simulink model "DolphinDrone_backup"  (R2024b)
settings: Solver=ode4  StartTime=0.0  StopTime=120  FixedStep=0.001  RelTol=1e-3
libraries: slpidlib x3, aerolibobsolete x1, simulink x1
settings Model: Creator=limchanyeong  LastModifiedBy=limchanyeong

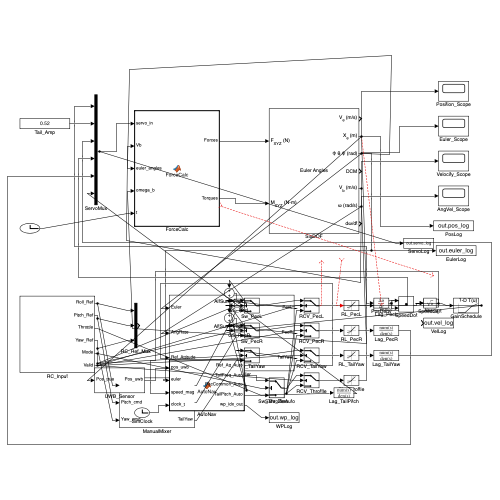
[thumbnail: Simulink's stored preview of the top-level diagram]
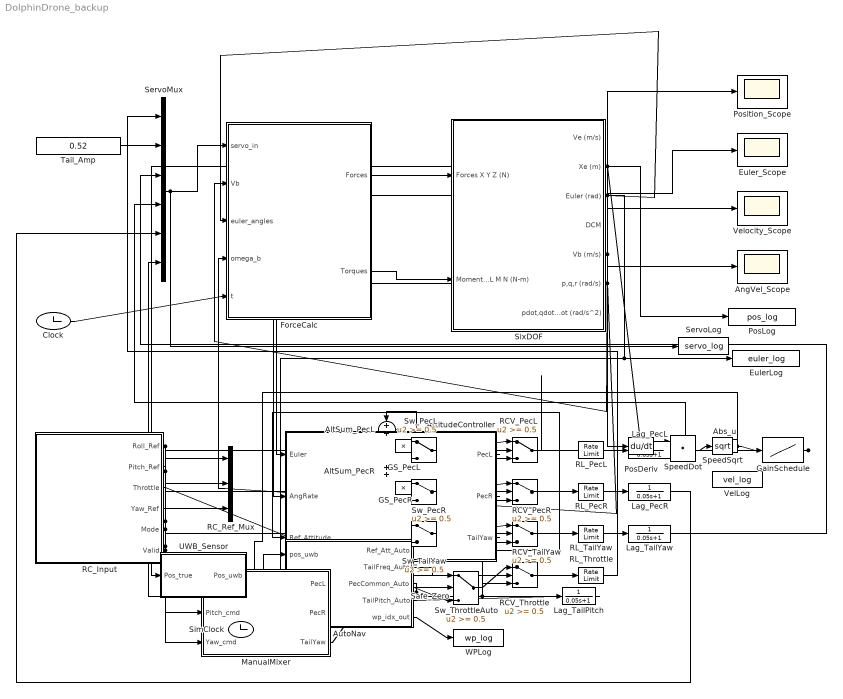
== system DolphinDrone_backup ==
  Abs_u : Abs  SaturateOnIntegerOverflow=off
  AltSum_PecL : Sum
  AltSum_PecR : Sum
  AngVel_Scope : Scope
  AttitudeController : Subsystem
  AutoNav : MATLAB Function  TreatAsAtomicUnit=on
  Clock : Clock
  EulerLog : ToWorkspace  VariableName=euler_log  SaveFormat=Timeseries  SampleTime=-1
  Euler_Scope : Scope
  ForceCalc : MATLAB Function  TreatAsAtomicUnit=on
  GS_PecL : Product
  GS_PecR : Product
  GainSchedule : Lookup_n-D  NumberOfTableDimensions=1  BreakpointsForDimension1=[0, 0.4, 0.8, 1.1]  Table=[0, 0, 0.7, 1]  InternalRulePriority=Speed  RndMeth=Simplest
  Lag_PecL : TransferFcn  Denominator=[0.05 1]
  Lag_PecR : TransferFcn  Denominator=[0.05 1]
  Lag_TailPitch : TransferFcn  Denominator=[0.05 1]
  Lag_TailYaw : TransferFcn  Denominator=[0.05 1]
  ManualMixer : Subsystem
  PosDeriv : Derivative
  PosLog : ToWorkspace  VariableName=pos_log  SaveFormat=Timeseries  SampleTime=-1
  Position_Scope : Scope
  RCV_PecL : Switch  Threshold=0.5  SaturateOnIntegerOverflow=off  InputSameDT=off
  RCV_PecR : Switch  Threshold=0.5  SaturateOnIntegerOverflow=off  InputSameDT=off
  RCV_TailYaw : Switch  Threshold=0.5  SaturateOnIntegerOverflow=off  InputSameDT=off
  RCV_Throttle : Switch  Threshold=0.5  SaturateOnIntegerOverflow=off  InputSameDT=off
  RC_Input : Subsystem
  RC_Ref_Mux : Mux  Inputs=3
  RL_PecL : RateLimiter  RisingSlewLimit=10  FallingSlewLimit=-10  SampleTimeMode=inherited
  RL_PecR : RateLimiter  RisingSlewLimit=10  FallingSlewLimit=-10  SampleTimeMode=inherited
  RL_TailYaw : RateLimiter  RisingSlewLimit=10  FallingSlewLimit=-10  SampleTimeMode=inherited
  RL_Throttle : RateLimiter  RisingSlewLimit=5  FallingSlewLimit=-5  SampleTimeMode=inherited
  Safe_Zero : Constant  Value=0
  ServoLog : ToWorkspace  VariableName=servo_log  SaveFormat=Timeseries  SampleTime=-1
  ServoMux : Mux  Inputs=6
  SimClock : Clock
  SixDOF : Subsystem  mask(6DOF EA Bridge){xme_0=[0,0,-1.5], Vm_0=[0, 0, 0], eul_0=[0,0,0], pm_0=[0, 0, 0], Mass=0.278269, Inertia=[0.006957 0 0; 0 0.059132 0; 0 0 0.059132]}
      mask prompts: xme_0 "Initial position in inertial axes [Xe,Ye,Ze] (m):"; Vm_0 "Initial velocity in body axes [U,v,w] (m/s):"; eul_0 "Initial Euler orientation [roll, pitch, yaw] (rad):"; pm_0 "Initial body rotation rates [p,q,r] (rad/s):"; Mass "Mass (kg):"; Inertia "Inertia matrix (kg.m^2):"
      mask help:
      | Block to bridge changes from version 1.0 and 1.0.1 to version 1.5.  Please consider updating your model.
      |
      | Integrate the six-degrees-of-freedom equations of motion using an Euler angle representation for the orientation of the body in space.
      mask Help: eval('asbhelp(''sixdof_euler_angles'')');
      mask Display:
      | port_label('input',1,'F_{XYZ} (N)','texmode','on');
      | port_label('input',2,'M_{XYZ} (N-m)','texmode','on');
      | port_label('output',1,'V_e (m/s)','texmode','on');
      | port_label('output',2,'X_e (m)','texmode','on');
      | port_label('output',3,'\phi \theta \psi (rad)','texmode','on');
      | port_label('output',4,'DCM','texmode','on');
      | port_label('output',5,'V_b (m/s)','texmode','on');
      | port_label('output',6,'\omega (rad/s)','texmode','on');
      | port_label('output',7,'d\omega/dt','texmode','on');
      | disp('Euler Angles')
  SpeedDot : DotProduct  OutDataTypeStr=Inherit: Inherit via internal rule
  SpeedSqrt : Sqrt
  Sw_PecL : Switch  Threshold=0.5  SaturateOnIntegerOverflow=off  InputSameDT=off
  Sw_PecR : Switch  Threshold=0.5  SaturateOnIntegerOverflow=off  InputSameDT=off
  Sw_TailYaw : Switch  Threshold=0.5  SaturateOnIntegerOverflow=off  InputSameDT=off
  Sw_ThrottleAuto : Switch  Threshold=0.5  SaturateOnIntegerOverflow=off  InputSameDT=off
  Tail_Amp : Constant  Value=0.52
  UWB_Sensor : Subsystem
  VelLog : ToWorkspace  VariableName=vel_log  SaveFormat=Timeseries  SampleTime=-1
  Velocity_Scope : Scope
  WPLog : ToWorkspace  VariableName=wp_log  SaveFormat=Timeseries  SampleTime=-1
  wires:
  Tail_Amp/1 -> ServoMux/2
  ServoMux/1 -> ForceCalc/1(servo_in), ServoLog/1
  Clock/1 -> ForceCalc/5(t)
  ForceCalc/1(Forces) -> SixDOF/1(Forces X Y Z (N))
  ForceCalc/2(Torques) -> SixDOF/2(Moments L M N (N-m))
  SixDOF/5(Vb (m/s)) -> ForceCalc/2(Vb), Velocity_Scope/1
  SixDOF/3(Euler (rad)) -> EulerLog/1, AutoNav/2(euler), ForceCalc/3(euler_angles), Euler_Scope/1, AttitudeController/1(Euler)
  SixDOF/6(p,q,r (rad/s)) -> ForceCalc/4(omega_b), AngVel_Scope/1, AttitudeController/2(AngRate)
  SixDOF/2(Xe (m)) -> Position_Scope/1, PosLog/1, PosDeriv/1, UWB_Sensor/1(Pos_true)
  RC_Input/1(Roll_Ref) -> RC_Ref_Mux/1, ManualMixer/1(Roll_cmd)
  RC_Input/2(Pitch_Ref) -> RC_Ref_Mux/2, ManualMixer/2(Pitch_cmd)
  RC_Input/4(Yaw_Ref) -> RC_Ref_Mux/3, ManualMixer/3(Yaw_cmd)
  RC_Input/5(Mode) -> Sw_PecL/2, Sw_PecR/2, Sw_TailYaw/2, Sw_ThrottleAuto/2
  ManualMixer/1(PecL) -> Sw_PecL/3
  ManualMixer/2(PecR) -> Sw_PecR/3
  ManualMixer/3(TailYaw) -> Sw_TailYaw/3
  Sw_PecL/1 -> RCV_PecL/1
  RC_Input/6(Valid) -> RCV_PecL/2, RCV_PecR/2, RCV_TailYaw/2, RCV_Throttle/2
  Safe_Zero/1 -> RCV_PecL/3, RCV_PecR/3, RCV_TailYaw/3, RCV_Throttle/3
  Sw_PecR/1 -> RCV_PecR/1
  Sw_TailYaw/1 -> RCV_TailYaw/1
  RC_Input/3(Throttle) -> Sw_ThrottleAuto/3
  RL_PecL/1 -> Lag_PecL/1
  Lag_PecL/1 -> ServoMux/4
  RCV_PecR/1 -> RL_PecR/1
  RL_PecR/1 -> Lag_PecR/1
  Lag_PecR/1 -> ServoMux/5
  RCV_TailYaw/1 -> RL_TailYaw/1
  RL_TailYaw/1 -> Lag_TailYaw/1
  Lag_TailYaw/1 -> ServoMux/3
  RCV_Throttle/1 -> RL_Throttle/1
  RL_Throttle/1 -> ServoMux/1
  GainSchedule/1 -> GS_PecL/2, GS_PecR/2
  ? -> ?
  AttitudeController/3(TailYaw) -> Sw_TailYaw/1
  Abs_u/1 -> GainSchedule/1
  RCV_PecL/1 -> ?
  ? -> RL_PecL/1
  PosDeriv/1 -> SpeedDot/1, SpeedDot/2
  SpeedDot/1 -> SpeedSqrt/1
  SpeedSqrt/1 -> Abs_u/1, AutoNav/3(speed_mag)
  UWB_Sensor/1(Pos_uwb) -> AutoNav/1(pos_uwb)
  SimClock/1 -> AutoNav/4(clock_t)
  AutoNav/2(TailFreq_Auto) -> Sw_ThrottleAuto/1
  AutoNav/1(Ref_Att_Auto) -> AttitudeController/3(Ref_Attitude)
  Sw_ThrottleAuto/1 -> RCV_Throttle/1
  AttitudeController/1(PecL) -> GS_PecL/1
  AttitudeController/2(PecR) -> GS_PecR/1
  GS_PecL/1 -> AltSum_PecL/1
  AutoNav/3(PecCommon_Auto) -> AltSum_PecL/2, AltSum_PecR/2
  AltSum_PecL/1 -> Sw_PecL/1
  GS_PecR/1 -> AltSum_PecR/1
  AltSum_PecR/1 -> Sw_PecR/1
  AutoNav/4(TailPitch_Auto) -> Lag_TailPitch/1
  Lag_TailPitch/1 -> ServoMux/6
  AutoNav/5(wp_idx_out) -> WPLog/1

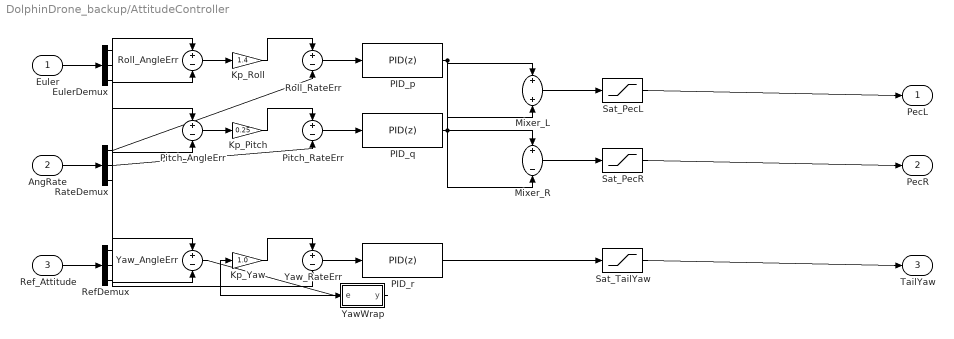
== system DolphinDrone_backup/AttitudeController ==
  Euler : Inport
  AngRate : Inport  Port=2
  Ref_Attitude : Inport  Port=3
  EulerDemux : Demux  Outputs=3
  Kp_Pitch : Gain  Gain=0.25
  Kp_Roll : Gain  Gain=1.4
  Kp_Yaw : Gain  Gain=1.0
  Mixer_L : Sum
  Mixer_R : Sum  Inputs=+-
  PID_p : slpidlib/PID Controller  Controller=PID  Form=Parallel  TimeDomain=Discrete-time  UseExternalTs=off  SampleTime=0.01  IntegratorMethod=Forward Euler  FilterMethod=Forward Euler  ControllerParametersSource=internal  P=0.3  I=0.01  UseKiTs=off  D=0.1  UseExternalDerivativeSource=off  N=100  UseFilter=on  TunerSelectOption=Transfer Function Based (PID Tuner App)  InitialConditionSource=internal  InitialConditionForIntegrator=0  InitialConditionForFilter=0  DifferentiatorICPrevScaledInput=0  ExternalReset=none  TrackingMode=off  Kt=1  LimitOutput=off  SatLimitsSource=internal  UpperSaturationLimit=0.6  LowerSaturationLimit=-0.6  LinearizeAsGain=off  AntiWindupMode=clamping  Kb=1  LimitIntegrator=off  UpperIntegratorSaturationLimit=inf  LowerIntegratorSaturationLimit=-inf  POutMin=[]  POutMax=[]  IOutMin=[]  IOutMax=[]  DOutMin=[]  DOutMax=[]  NOutMin=[]  NOutMax=[]  SumOutMin=[]  SumOutMax=[]  SaturationOutMin=[]  SaturationOutMax=[]  PParamMin=[]  PParamMax=[]  IParamMin=[]  IParamMax=[]  DParamMin=[]  DParamMax=[]  NParamMin=[]  NParamMax=[]  KbParamMin=[]  KbParamMax=[]  KtParamMin=[]  KtParamMax=[]  KbOutMin=[]  KbOutMax=[]  KtOutMin=[]  KtOutMax=[]  IntegratorOutMin=[]  IntegratorOutMax=[]  FilterOutMin=[]  FilterOutMax=[]  SumI1OutMin=[]  SumI1OutMax=[]  SumI2OutMin=[]  SumI2OutMax=[]  SumI3OutMin=[]  SumI3OutMax=[]  SumI4OutMin=[]  SumI4OutMax=[]  SumDOutMin=[]  SumDOutMax=[]  DifferentiatorOutMin=[]  DifferentiatorOutMax=[]  FilterDiffOutCoefMin=[]  FilterDiffOutCoefMax=[]  ReciprocalOutMin=[]  ReciprocalOutMax=[]  SumDenOutMin=[]  SumDenOutMax=[]  SumNumOutMin=[]  SumNumOutMax=[]  DivideOutMin=[]  DivideOutMax=[]  UdiffTsProdOutMin=[]  UdiffTsProdOutMax=[]  NTsProdOutMin=[]  NTsProdOutMax=[]  UintegralTsProdOutMin=[]  UintegralTsProdOutMax=[]  UngainTsProdOutMin=[]  UngainTsProdOutMax=[]  ClampingZeroOutDataTypeStr=Inherit: Inherit via back propagation  ClampingZeroOutMin=[]  ClampingZeroOutMax=[]  FilterDenConstantOutDataTypeStr=Inherit: Inherit via back propagation  FilterDenConstantOutMin=[]  FilterDenConstantOutMax=[]  PCopyOutDataTypeStr=Inherit: Inherit via back propagation  PCopyOutMin=[]  PCopyOutMax=[]  NCopyOutDataTypeStr=Inherit: Inherit via back propagation  NCopyOutMin=[]  NCopyOutMax=[]  IntegratorContinuousStateAttributes=''  IntegratorStateMustResolveToSignalObject=off  IntegratorRTWStateStorageClass=Auto  FilterContinuousStateAttributes=''  FilterStateMustResolveToSignalObject=off  FilterRTWStateStorageClass=Auto  ParallelPVariant=InternalParameters  IdealPVariant=Disabled  IVariant=InternalParameters  DVariant=InternalParameters  IntegratorVariant=Discrete  SatVariant=Disabled  AWVariant=Passthrough  PCopyVariant=Disabled  TRVariant=Disabled  FdbkBlocksVariant=Forward  IdealPFdbkVariant=Disabled  SatFdbkVariant=Disabled  DerivativeFilterVariant=ForwardEulerFilter  NVariant=InternalParameters  NCopyVariant=Disabled  FilterICVariant=InternalICsFilter  IntegratorICVariant=InternalICs  ExternalResetVariant=Disabled  TRSumVariant=Passthrough  SumFdbkVariant=Disabled  SumVariant=Sum_PID  TsampFilterVariant=InternalTs  TsampNgainVariant=Passthrough  TsampIntegralVariant=Disabled_SignalSpec  ExternalSaturationOutDataTypeStr=Inherit: Same as second input  DerivativeSourceVariant=ErrorSignal  PreIntVariant=InternalPreInt
      settings: LibrarySourceBlock=simulink/Discrete/Discrete PID Controller
  PID_q : slpidlib/PID Controller  Controller=PID  Form=Parallel  TimeDomain=Discrete-time  UseExternalTs=off  SampleTime=0.01  IntegratorMethod=Forward Euler  FilterMethod=Forward Euler  ControllerParametersSource=internal  P=0.20  I=0  UseKiTs=off  D=0.02  UseExternalDerivativeSource=off  N=100  UseFilter=on  TunerSelectOption=Transfer Function Based (PID Tuner App)  InitialConditionSource=internal  InitialConditionForIntegrator=0  InitialConditionForFilter=0  DifferentiatorICPrevScaledInput=0  ExternalReset=none  TrackingMode=off  Kt=1  LimitOutput=off  SatLimitsSource=internal  UpperSaturationLimit=0.6  LowerSaturationLimit=-0.6  LinearizeAsGain=off  AntiWindupMode=clamping  Kb=1  LimitIntegrator=off  UpperIntegratorSaturationLimit=inf  LowerIntegratorSaturationLimit=-inf  POutMin=[]  POutMax=[]  IOutMin=[]  IOutMax=[]  DOutMin=[]  DOutMax=[]  NOutMin=[]  NOutMax=[]  SumOutMin=[]  SumOutMax=[]  SaturationOutMin=[]  SaturationOutMax=[]  PParamMin=[]  PParamMax=[]  IParamMin=[]  IParamMax=[]  DParamMin=[]  DParamMax=[]  NParamMin=[]  NParamMax=[]  KbParamMin=[]  KbParamMax=[]  KtParamMin=[]  KtParamMax=[]  KbOutMin=[]  KbOutMax=[]  KtOutMin=[]  KtOutMax=[]  IntegratorOutMin=[]  IntegratorOutMax=[]  FilterOutMin=[]  FilterOutMax=[]  SumI1OutMin=[]  SumI1OutMax=[]  SumI2OutMin=[]  SumI2OutMax=[]  SumI3OutMin=[]  SumI3OutMax=[]  SumI4OutMin=[]  SumI4OutMax=[]  SumDOutMin=[]  SumDOutMax=[]  DifferentiatorOutMin=[]  DifferentiatorOutMax=[]  FilterDiffOutCoefMin=[]  FilterDiffOutCoefMax=[]  ReciprocalOutMin=[]  ReciprocalOutMax=[]  SumDenOutMin=[]  SumDenOutMax=[]  SumNumOutMin=[]  SumNumOutMax=[]  DivideOutMin=[]  DivideOutMax=[]  UdiffTsProdOutMin=[]  UdiffTsProdOutMax=[]  NTsProdOutMin=[]  NTsProdOutMax=[]  UintegralTsProdOutMin=[]  UintegralTsProdOutMax=[]  UngainTsProdOutMin=[]  UngainTsProdOutMax=[]  ClampingZeroOutDataTypeStr=Inherit: Inherit via back propagation  ClampingZeroOutMin=[]  ClampingZeroOutMax=[]  FilterDenConstantOutDataTypeStr=Inherit: Inherit via back propagation  FilterDenConstantOutMin=[]  FilterDenConstantOutMax=[]  PCopyOutDataTypeStr=Inherit: Inherit via back propagation  PCopyOutMin=[]  PCopyOutMax=[]  NCopyOutDataTypeStr=Inherit: Inherit via back propagation  NCopyOutMin=[]  NCopyOutMax=[]  IntegratorContinuousStateAttributes=''  IntegratorStateMustResolveToSignalObject=off  IntegratorRTWStateStorageClass=Auto  FilterContinuousStateAttributes=''  FilterStateMustResolveToSignalObject=off  FilterRTWStateStorageClass=Auto  ParallelPVariant=InternalParameters  IdealPVariant=Disabled  IVariant=InternalParameters  DVariant=InternalParameters  IntegratorVariant=Discrete  SatVariant=Disabled  AWVariant=Passthrough  PCopyVariant=Disabled  TRVariant=Disabled  FdbkBlocksVariant=Forward  IdealPFdbkVariant=Disabled  SatFdbkVariant=Disabled  DerivativeFilterVariant=ForwardEulerFilter  NVariant=InternalParameters  NCopyVariant=Disabled  FilterICVariant=InternalICsFilter  IntegratorICVariant=InternalICs  ExternalResetVariant=Disabled  TRSumVariant=Passthrough  SumFdbkVariant=Disabled  SumVariant=Sum_PID  TsampFilterVariant=InternalTs  TsampNgainVariant=Passthrough  TsampIntegralVariant=Disabled_SignalSpec  ExternalSaturationOutDataTypeStr=Inherit: Same as second input  DerivativeSourceVariant=ErrorSignal  PreIntVariant=InternalPreInt
      settings: LibrarySourceBlock=simulink/Discrete/Discrete PID Controller
  PID_r : slpidlib/PID Controller  Controller=PID  Form=Parallel  TimeDomain=Discrete-time  UseExternalTs=off  SampleTime=0.01  IntegratorMethod=Forward Euler  FilterMethod=Forward Euler  ControllerParametersSource=internal  P=0.2  I=0.02  UseKiTs=off  D=0.03  UseExternalDerivativeSource=off  N=100  UseFilter=on  TunerSelectOption=Transfer Function Based (PID Tuner App)  InitialConditionSource=internal  InitialConditionForIntegrator=0  InitialConditionForFilter=0  DifferentiatorICPrevScaledInput=0  ExternalReset=none  TrackingMode=off  Kt=1  LimitOutput=off  SatLimitsSource=internal  UpperSaturationLimit=0.52  LowerSaturationLimit=-0.52  LinearizeAsGain=off  AntiWindupMode=clamping  Kb=1  LimitIntegrator=off  UpperIntegratorSaturationLimit=inf  LowerIntegratorSaturationLimit=-inf  POutMin=[]  POutMax=[]  IOutMin=[]  IOutMax=[]  DOutMin=[]  DOutMax=[]  NOutMin=[]  NOutMax=[]  SumOutMin=[]  SumOutMax=[]  SaturationOutMin=[]  SaturationOutMax=[]  PParamMin=[]  PParamMax=[]  IParamMin=[]  IParamMax=[]  DParamMin=[]  DParamMax=[]  NParamMin=[]  NParamMax=[]  KbParamMin=[]  KbParamMax=[]  KtParamMin=[]  KtParamMax=[]  KbOutMin=[]  KbOutMax=[]  KtOutMin=[]  KtOutMax=[]  IntegratorOutMin=[]  IntegratorOutMax=[]  FilterOutMin=[]  FilterOutMax=[]  SumI1OutMin=[]  SumI1OutMax=[]  SumI2OutMin=[]  SumI2OutMax=[]  SumI3OutMin=[]  SumI3OutMax=[]  SumI4OutMin=[]  SumI4OutMax=[]  SumDOutMin=[]  SumDOutMax=[]  DifferentiatorOutMin=[]  DifferentiatorOutMax=[]  FilterDiffOutCoefMin=[]  FilterDiffOutCoefMax=[]  ReciprocalOutMin=[]  ReciprocalOutMax=[]  SumDenOutMin=[]  SumDenOutMax=[]  SumNumOutMin=[]  SumNumOutMax=[]  DivideOutMin=[]  DivideOutMax=[]  UdiffTsProdOutMin=[]  UdiffTsProdOutMax=[]  NTsProdOutMin=[]  NTsProdOutMax=[]  UintegralTsProdOutMin=[]  UintegralTsProdOutMax=[]  UngainTsProdOutMin=[]  UngainTsProdOutMax=[]  ClampingZeroOutDataTypeStr=Inherit: Inherit via back propagation  ClampingZeroOutMin=[]  ClampingZeroOutMax=[]  FilterDenConstantOutDataTypeStr=Inherit: Inherit via back propagation  FilterDenConstantOutMin=[]  FilterDenConstantOutMax=[]  PCopyOutDataTypeStr=Inherit: Inherit via back propagation  PCopyOutMin=[]  PCopyOutMax=[]  NCopyOutDataTypeStr=Inherit: Inherit via back propagation  NCopyOutMin=[]  NCopyOutMax=[]  IntegratorContinuousStateAttributes=''  IntegratorStateMustResolveToSignalObject=off  IntegratorRTWStateStorageClass=Auto  FilterContinuousStateAttributes=''  FilterStateMustResolveToSignalObject=off  FilterRTWStateStorageClass=Auto  ParallelPVariant=InternalParameters  IdealPVariant=Disabled  IVariant=InternalParameters  DVariant=InternalParameters  IntegratorVariant=Discrete  SatVariant=Disabled  AWVariant=Passthrough  PCopyVariant=Disabled  TRVariant=Disabled  FdbkBlocksVariant=Forward  IdealPFdbkVariant=Disabled  SatFdbkVariant=Disabled  DerivativeFilterVariant=ForwardEulerFilter  NVariant=InternalParameters  NCopyVariant=Disabled  FilterICVariant=InternalICsFilter  IntegratorICVariant=InternalICs  ExternalResetVariant=Disabled  TRSumVariant=Passthrough  SumFdbkVariant=Disabled  SumVariant=Sum_PID  TsampFilterVariant=InternalTs  TsampNgainVariant=Passthrough  TsampIntegralVariant=Disabled_SignalSpec  ExternalSaturationOutDataTypeStr=Inherit: Same as second input  DerivativeSourceVariant=ErrorSignal  PreIntVariant=InternalPreInt
      settings: LibrarySourceBlock=simulink/Discrete/Discrete PID Controller
  Pitch_AngleErr : Sum  Inputs=+-
  Pitch_RateErr : Sum  Inputs=+-
  RateDemux : Demux  Outputs=3
  RefDemux : Demux  Outputs=3
  Roll_AngleErr : Sum  Inputs=+-
  Roll_RateErr : Sum  Inputs=+-
  Sat_PecL : Saturate  UpperLimit=0.61  LowerLimit=-0.61
  Sat_PecR : Saturate  UpperLimit=0.61  LowerLimit=-0.61
  Sat_TailYaw : Saturate  UpperLimit=0.785  LowerLimit=-0.785
  YawWrap : MATLAB Function  TreatAsAtomicUnit=on
  Yaw_AngleErr : Sum  Inputs=+-
  Yaw_RateErr : Sum  Inputs=+-
  PecL : Outport
  PecR : Outport  Port=2
  TailYaw : Outport  Port=3
  wires:
  Euler/1 -> EulerDemux/1
  AngRate/1 -> RateDemux/1
  Ref_Attitude/1 -> RefDemux/1
  RefDemux/1 -> Roll_AngleErr/1
  EulerDemux/1 -> Roll_AngleErr/2
  Roll_AngleErr/1 -> Kp_Roll/1
  Kp_Roll/1 -> Roll_RateErr/1
  RateDemux/1 -> Roll_RateErr/2
  Roll_RateErr/1 -> PID_p/1
  RefDemux/2 -> Pitch_AngleErr/1
  EulerDemux/2 -> Pitch_AngleErr/2
  Pitch_AngleErr/1 -> Kp_Pitch/1
  Kp_Pitch/1 -> Pitch_RateErr/1
  RateDemux/2 -> Pitch_RateErr/2
  Pitch_RateErr/1 -> PID_q/1
  RefDemux/3 -> Yaw_AngleErr/1
  EulerDemux/3 -> Yaw_AngleErr/2
  Kp_Yaw/1 -> Yaw_RateErr/1
  RateDemux/3 -> Yaw_RateErr/2
  Yaw_RateErr/1 -> PID_r/1
  PID_q/1 -> Mixer_L/1, Mixer_R/1
  PID_p/1 -> Mixer_L/2, Mixer_R/2
  Mixer_L/1 -> Sat_PecL/1
  Sat_PecL/1 -> PecL/1
  Mixer_R/1 -> Sat_PecR/1
  Sat_PecR/1 -> PecR/1
  PID_r/1 -> Sat_TailYaw/1
  Sat_TailYaw/1 -> TailYaw/1
  Yaw_AngleErr/1 -> YawWrap/1(e)
  YawWrap/1(y) -> Kp_Yaw/1

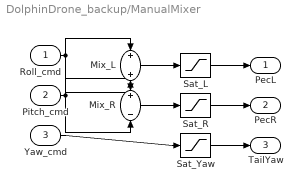
== system DolphinDrone_backup/ManualMixer ==
  Roll_cmd : Inport
  Pitch_cmd : Inport  Port=2
  Yaw_cmd : Inport  Port=3
  Mix_L : Sum
  Mix_R : Sum  Inputs=+-
  Sat_L : Saturate  UpperLimit=0.61  LowerLimit=-0.61
  Sat_R : Saturate  UpperLimit=0.61  LowerLimit=-0.61
  Sat_Yaw : Saturate  UpperLimit=0.52  LowerLimit=-0.52
  PecL : Outport
  PecR : Outport  Port=2
  TailYaw : Outport  Port=3
  wires:
  Pitch_cmd/1 -> Mix_L/1, Mix_R/1
  Roll_cmd/1 -> Mix_L/2, Mix_R/2
  Mix_L/1 -> Sat_L/1
  Mix_R/1 -> Sat_R/1
  Yaw_cmd/1 -> Sat_Yaw/1
  Sat_L/1 -> PecL/1
  Sat_R/1 -> PecR/1
  Sat_Yaw/1 -> TailYaw/1

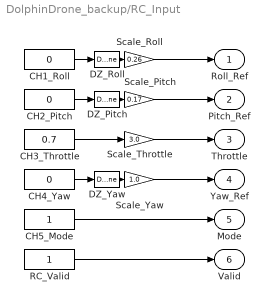
== system DolphinDrone_backup/RC_Input ==
  CH1_Roll : Constant  Value=0
  CH2_Pitch : Constant  Value=0
  CH3_Throttle : Constant  Value=0.7
  CH4_Yaw : Constant  Value=0
  CH5_Mode : Constant
  DZ_Pitch : DeadZone  LowerValue=-0.05  UpperValue=0.05
  DZ_Roll : DeadZone  LowerValue=-0.05  UpperValue=0.05
  DZ_Yaw : DeadZone  LowerValue=-0.05  UpperValue=0.05
  RC_Valid : Constant
  Scale_Pitch : Gain  Gain=0.17
  Scale_Roll : Gain  Gain=0.26
  Scale_Throttle : Gain  Gain=3.0
  Scale_Yaw : Gain  Gain=1.0
  Roll_Ref : Outport
  Pitch_Ref : Outport  Port=2
  Throttle : Outport  Port=3
  Yaw_Ref : Outport  Port=4
  Mode : Outport  Port=5
  Valid : Outport  Port=6
  wires:
  CH3_Throttle/1 -> Scale_Throttle/1
  Scale_Roll/1 -> Roll_Ref/1
  Scale_Pitch/1 -> Pitch_Ref/1
  Scale_Throttle/1 -> Throttle/1
  Scale_Yaw/1 -> Yaw_Ref/1
  CH5_Mode/1 -> Mode/1
  CH1_Roll/1 -> DZ_Roll/1
  DZ_Roll/1 -> Scale_Roll/1
  CH2_Pitch/1 -> DZ_Pitch/1
  DZ_Pitch/1 -> Scale_Pitch/1
  CH4_Yaw/1 -> DZ_Yaw/1
  DZ_Yaw/1 -> Scale_Yaw/1
  RC_Valid/1 -> Valid/1

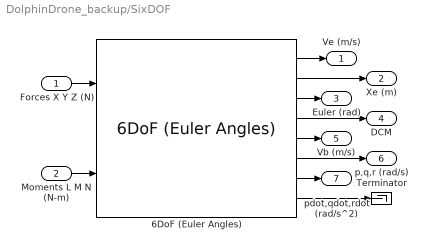
== system DolphinDrone_backup/SixDOF ==
  Forces X Y Z (N) : Inport  OutDataTypeStr=double
  Moments L M N (N-m) : Inport  Port=2  OutDataTypeStr=double
  6DoF (Euler Angles) : aerolibobsolete/6DoF (Euler Angles)  units=Metric (MKS)  mtype=Fixed  rep=Euler Angles  xme_0=xme_0  Vm_0=Vm_0  eul_0=eul_0  pm_0=pm_0  mass_0=Mass  mass_e=0.5  mass_f=2.0  inertia=Inertia  inertia_e=eye(3)  inertia_f=2*eye(3)  k_quat=1.0
  Terminator : Terminator
  Ve (m/s) : Outport
  Xe (m) : Outport  Port=2
  Euler (rad) : Outport  Port=3
  DCM : Outport  Port=4
  Vb (m/s) : Outport  Port=5
  p,q,r (rad/s) : Outport  Port=6
  pdot,qdot,rdot (rad/s^2) : Outport  Port=7
  wires:
  6DoF (Euler Angles)/8 -> Terminator/1
  6DoF (Euler Angles)/1 -> Ve (m/s)/1
  6DoF (Euler Angles)/2 -> Xe (m)/1
  Forces X Y Z (N)/1 -> 6DoF (Euler Angles)/1
  6DoF (Euler Angles)/3 -> Euler (rad)/1
  6DoF (Euler Angles)/4 -> DCM/1
  6DoF (Euler Angles)/5 -> Vb (m/s)/1
  6DoF (Euler Angles)/6 -> p,q,r (rad/s)/1
  Moments L M N (N-m)/1 -> 6DoF (Euler Angles)/2
  6DoF (Euler Angles)/7 -> pdot,qdot,rdot (rad/s^2)/1

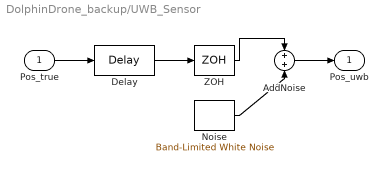
== system DolphinDrone_backup/UWB_Sensor ==
  Pos_true : Inport
  AddNoise : Sum
  Delay : TransportDelay  DelayTime=0.10
  Noise : simulink/Sources/Band-Limited White Noise  Cov=[0.08^2, 0.08^2, 0.12^2]  Ts=0.1  seed=[1 2 3]
  ZOH : ZeroOrderHold  SampleTime=0.1
  Pos_uwb : Outport
  wires:
  ? -> ?
  Pos_true/1 -> Delay/1
  Delay/1 -> ZOH/1
  ZOH/1 -> AddNoise/1
  Noise/1 -> AddNoise/2
  AddNoise/1 -> Pos_uwb/1

== matlab function DolphinDrone_backup/AutoNav ==
  settings: updateMethod=DISCRETE  sampleTime=0.1
  data: pos_uwb input; Ref_Att_Auto output; euler input; speed_mag input; clock_t input; TailFreq_Auto output; PecCommon_Auto output; TailPitch_Auto output; wp_idx_out output
function [Ref_Att_Auto, TailFreq_Auto, PecCommon_Auto, TailPitch_Auto, wp_idx_out] = AutoNav(pos_uwb, euler, speed_mag, clock_t)
%#codegen
%% AutoNav: 위치 제어기 (LOS + 미리 꺾기)
%%
%% 핵심: 현재 WP에 가까워지면 다음 WP 방향을 미리 블렌딩
%%       → 코너에서 자연스럽게 턴 시작

%% ========== 파라미터 ==========
WP = [ 0,  0, -1.5;
       5,  0, -1.5;
       5,  5, -1.5;
       0,  5, -1.5;
       0,  0, -1.5];
N_wp = 5;

% WP 전환
R_switch = 0.5;          % WP 전환: 가까이 가서 전환
R_blend = 2.0;           % 미리 꺾기: 일찍 시작

% LOS
T_look = 0.6;
L_look_min = 0.4;
L_look_max = 1.0;
K_ct = 1.5;
psi_rate_max = 55 * pi/180;  % 빠른 턴

% Speed
u_cruise = 0.8;        % 순항 낮춤
u_corner = 0.3;        % 코너에서 거의 멈춤
Kp_u = 0.8;
Ki_u = 0.15;
freq_min = 0.5;
freq_max = 3.0;

% Altitude - tail pitch
Kp_h_tail = 0.15;
tail_pitch_max = 0.25;
rho_air = 1.225;
S_tail_area = 0.02;
C_T = 0.30;
tail_amp_nom = 0.52;
F_neg_buoy = 0.0005 * 9.81;

% Altitude - pec common
Kp_h_pec = 0.03;
pec_common_max = 0.10;
S_pec = 0.01;
CL_alpha = 2*pi;

% Bank
K_bank = 0.10;
phi_max = 3 * pi/180;

%% ========== Persistent ==========
persistent wp_idx u_integral prev_psi_ref prev_height
dt = 0.1;

if isempty(wp_idx) || clock_t < dt
    wp_idx = 1;
    u_integral = 0;
    prev_psi_ref = 0;
    prev_height = 1.5;
end

%% ========== 상태 ==========
x = pos_uwb(1);  y = pos_uwb(2);  z = pos_uwb(3);
psi = euler(3);
height = -z;
u_meas = max(speed_mag, 0.0);

%% ========== 1. Waypoint Manager ==========
% 현재 목표 WP
tgt_x = WP(wp_idx, 1);
tgt_y = WP(wp_idx, 2);
dist_to_wp = sqrt((x - tgt_x)^2 + (y - tgt_y)^2);

% WP 전환
if dist_to_wp < R_switch && wp_idx < N_wp
    wp_idx = wp_idx + 1;
end

% 현재/다음 WP
tgt_x = WP(wp_idx, 1);
tgt_y = WP(wp_idx, 2);
tgt_z = WP(wp_idx, 3);
h_ref = -tgt_z;
dist_to_wp = sqrt((x - tgt_x)^2 + (y - tgt_y)^2);

%% ========== 2. Guidance: 미리 꺾기 + WP 방향 ==========
% 현재 WP로의 heading
psi_to_current = atan2(tgt_y - y, tgt_x - x);

% 다음 WP가 있으면 블렌딩
if wp_idx < N_wp && dist_to_wp < R_blend
    next_x = WP(wp_idx + 1, 1);
    next_y = WP(wp_idx + 1, 2);
    psi_to_next = atan2(next_y - y, next_x - x);

    sigma = max(min((R_blend - dist_to_wp) / R_blend, 1.0), 0.0);
    alpha = 0.85 * (3*sigma^2 - 2*sigma^3);

    t1x = cos(psi_to_current); t1y = sin(psi_to_current);
    t2x = cos(psi_to_next);    t2y = sin(psi_to_next);
    dx_blend = (1-alpha)*t1x + alpha*t2x;
    dy_blend = (1-alpha)*t1y + alpha*t2y;
    psi_desired = atan2(dy_blend, dx_blend);
else
    psi_desired = psi_to_current;
end

% psi_ref rate limiting
psi_err_raw = atan2(sin(psi_desired - prev_psi_ref), cos(psi_desired - prev_psi_ref));
dpsi_cmd = max(min(psi_err_raw, psi_rate_max * dt), -psi_rate_max * dt);
psi_ref = prev_psi_ref + dpsi_cmd;
psi_ref = atan2(sin(psi_ref), cos(psi_ref));
prev_psi_ref = psi_ref;

% heading error
psi_err = atan2(sin(psi_ref - psi), cos(psi_ref - psi));

% 속도: 코너 접근 시 감속 (블렌딩 구간보다 넓게)
R_slow = R_blend + 1.0;  % 감속 시작 = 블렌딩보다 1m 먼저
if dist_to_wp < R_slow && wp_idx < N_wp
    u_ref = u_corner + (u_cruise - u_corner) * (dist_to_wp / R_slow);
else
    u_ref = u_cruise;
end

%% ========== 3. Speed Controller (PI) ==========
u_err = u_ref - u_meas;
u_integral = u_integral + u_err * dt;
u_integral = max(min(u_integral, 3.0), -1.0);
tail_freq = Kp_u * u_err + Ki_u * u_integral;
tail_freq = max(min(tail_freq, freq_max), freq_min);
tail_freq = max(tail_freq, 1.1);  % altitude floor

%% ========== 4. Altitude ==========
h_err = h_ref - height;
prev_height = height;

% Tail pitch (primary)
F_thr_est = rho_air * pi^2 * S_tail_area * tail_amp_nom^2 * tail_freq^2 * C_T;
F_thr_est = max(F_thr_est, 0.001);
tail_pitch_ff = -asin(min(max(F_neg_buoy / F_thr_est, -0.4), 0.4));
tail_pitch_fb = -(Kp_h_tail * h_err);
tail_pitch_cmd = tail_pitch_ff + tail_pitch_fb;
tail_pitch_cmd = max(min(tail_pitch_cmd, tail_pitch_max), -tail_pitch_max);

% Pec common (secondary)
u_eff = max(u_meas, 0.65);
pec_ff = F_neg_buoy / (rho_air * u_eff^2 * S_pec * CL_alpha) * 0.5;
pec_fb = Kp_h_pec * h_err;
pec_common = pec_ff + pec_fb;
pec_common = max(min(pec_common, pec_common_max), -pec_common_max);

%% ========== 5. Bank Turn ==========
phi_bank = K_bank * psi_err;
phi_bank = max(min(phi_bank, phi_max), -phi_max);
if u_meas < 0.7
    phi_bank = 0;
end

%% ========== 출력 ==========
Ref_Att_Auto = [phi_bank; 0; psi_ref];
TailFreq_Auto = tail_freq;
PecCommon_Auto = pec_common;
TailPitch_Auto = tail_pitch_cmd;
wp_idx_out = wp_idx;

end

== matlab function DolphinDrone_backup/ForceCalc ==
  data: servo_in input size=6; Forces output; Vb input; euler_angles input; omega_b input; t input; Torques output
function [Forces, Torques] = ForceCalc(servo_in, Vb, euler_angles, omega_b, t)
%#codegen
%% 돌고래 헬륨 드론 힘/토크 계산
%% MATLAB Function 블록에 이 코드를 복사-붙여넣기 하세요
%%
%% 입력:
%%   servo_in(5x1): [tail_freq, tail_amp, tail_yaw, pec_left, pec_right]
%%   Vb(3x1):       기체 좌표계 속도 [u, v, w]
%%   euler_angles(3x1): [phi, theta, psi]
%%   omega_b(3x1):  각속도 [p, q, r]
%%   t(1x1):        시간 [s]
%%
%% 출력:
%%   Forces(3x1):  기체 좌표계 합력 [Fx, Fy, Fz]
%%   Torques(3x1): 기체 좌표계 합토크 [L, M, N]

Forces = zeros(1,3);
Torques = zeros(1,3);

%% ========== 파라미터 ==========
rho_air = 1.225;    % 공기 밀도 [kg/m³]
rho_He  = 0.164;    % 헬륨 밀도 [kg/m³]
g       = 9.81;     % 중력 가속도 [m/s²]

% 기체 형상 / 정적 trim
body_length   = 2.0;    % [m]
body_max_diam = 0.50;   % [m] (재설계: 0.58→0.50)
a_semi = body_length / 2;
b_semi = body_max_diam / 2;
V_env  = (4/3) * pi * a_semi * b_semi^2;

m_neutral   = (rho_air - rho_He) * V_env;
buoy_margin = -0.0005;  % [kg], 약 -0.5 g 음성부력
m_total     = m_neutral - buoy_margin;

% 꼬리
S_tail  = 0.02;     % 꼬리 면적 [m²]
C_T     = 0.30;     % 추력계수
r_tail_x = -0.80;   % 꼬리 x위치 [m] (후방)
tail_freq_min = 0.5;
tail_freq_max = 3.0;
tail_amp_max  = 0.70;
tail_yaw_max  = 0.785;   % 45 deg

% 가슴지느러미
S_pec    = 0.01;    % 면적 [m²]
CL_alpha = 2*pi;    % 양력 기울기 [1/rad]
r_pec_y  = 0.25;    % y위치 [m]
r_pec_x  = 0.10;    % x위치 [m]
pec_delta_max   = 35*pi/180;
pec_alpha_stall = 15*pi/180;
pec_CL_max      = 1.20;
pec_V_min       = 0.05; % 저속 surrogate용 최소 유속 [m/s]

% 등지느러미 (고정, 수동 감쇠)
C_damp_yaw  = 0.005;
C_damp_roll = 0.003;

% 공기 항력
Cd    = 0.30;
S_ref = pi * b_semi^2;   % 정면 단면적 [m²]

% 부력-무게중심 오프셋
r_CB_CG = [0; 0; -0.05]; % CB가 CG보다 5cm 위 (NED z-down)

%% ========== 서보 입력 분리 ==========
tail_freq      = min(max(servo_in(1), tail_freq_min), tail_freq_max);
tail_amp       = min(max(servo_in(2), 0.0), tail_amp_max);
tail_yaw_cmd   = min(max(servo_in(3), -tail_yaw_max), tail_yaw_max);
pec_left       = min(max(servo_in(4), -pec_delta_max), pec_delta_max);
pec_right      = min(max(servo_in(5), -pec_delta_max), pec_delta_max);
tail_pitch_cmd = min(max(servo_in(6), -0.25), 0.25);  % 꼬리 상하 편향 [rad]

%% ========== 상태 변수 ==========
phi   = euler_angles(1);
theta = euler_angles(2);
psi   = euler_angles(3);

u = Vb(1); v = Vb(2); w = Vb(3);
V_mag = sqrt(u^2 + v^2 + w^2);

p = omega_b(1); q = omega_b(2); r = omega_b(3);

%% ========== 1. DCM (Earth → Body) ==========
cphi = cos(phi);  sphi = sin(phi);
cth  = cos(theta); sth = sin(theta);
cpsi = cos(psi);  spsi = sin(psi);

R = [ cth*cpsi,                 cth*spsi,                -sth;
      sphi*sth*cpsi-cphi*spsi,  sphi*sth*spsi+cphi*cpsi,  sphi*cth;
      cphi*sth*cpsi+sphi*spsi,  cphi*sth*spsi-sphi*cpsi,  cphi*cth];

%% ========== 2. 부력 (NED: Z 하향, 부력은 -Z) ==========
F_buoy_e = [0; 0; -(rho_air - rho_He) * V_env * g];
F_buoy_b = R * F_buoy_e;
T_buoy   = cross(r_CB_CG, F_buoy_b);

%% ========== 3. 중력 (NED: +Z 하향) ==========
F_grav_e = [0; 0; m_total * g];
F_grav_b = R * F_grav_e;

%% ========== 4. 꼬리 추진력 ==========
F_thr = rho_air * pi^2 * S_tail * tail_amp^2 * tail_freq^2 * C_T;

F_tail = [F_thr * cos(tail_yaw_cmd) * cos(tail_pitch_cmd);  % 전진
          F_thr * sin(tail_yaw_cmd);                         % 횡방향 (yaw)
          F_thr * cos(tail_yaw_cmd) * sin(tail_pitch_cmd)];  % 수직 (pitch)

% Yaw + Pitch 토크
T_tail = [0;
          -F_thr * sin(tail_pitch_cmd) * abs(r_tail_x);  % Pitch 모멘트
          F_thr * sin(tail_yaw_cmd) * abs(r_tail_x)];    % Yaw 모멘트

%% ========== 5. 가슴지느러미 ==========
% 정지 호버에서 양력이 생기지 않도록 전방 유속 기반으로 계산하되,
% 수치적으로 완전히 0이 되지 않게 작은 surrogate 유속을 둡니다.
V_pec = max(abs(u), pec_V_min);
q_pec = 0.5 * rho_air * V_pec^2;

alpha_pL = min(max(pec_left,  -pec_alpha_stall), pec_alpha_stall);
alpha_pR = min(max(pec_right, -pec_alpha_stall), pec_alpha_stall);
CL_pL = min(max(CL_alpha * alpha_pL, -pec_CL_max), pec_CL_max);
CL_pR = min(max(CL_alpha * alpha_pR, -pec_CL_max), pec_CL_max);

Fz_pec_L = -q_pec * S_pec * CL_pL; % body z-down, 음수는 upward
Fz_pec_R = -q_pec * S_pec * CL_pR;
Fz_pec = Fz_pec_L + Fz_pec_R;

% 좌: y=-r_pec_y, 우: y=+r_pec_y 로 가정한 모멘트
T_roll_pec  = r_pec_y * (Fz_pec_R - Fz_pec_L);
T_pitch_pec = -r_pec_x * Fz_pec;

%% ========== 6. 등지느러미 수동 감쇠 ==========
T_dorsal = [-C_damp_roll * p;    % Roll 감쇠
             0;                   % Pitch 무관
            -C_damp_yaw * r];     % Yaw 감쇠

%% ========== 7. 공기 항력 ==========
if V_mag > 0.001
    F_drag = -0.5 * rho_air * Cd * S_ref * V_mag * Vb;
else
    F_drag = zeros(3,1);
end

% 회전 감쇠
T_rot_damp = -0.001 * omega_b;

%% ========== 합산 ==========
Forces  = (F_buoy_b + F_grav_b + F_tail + [0; 0; Fz_pec] + F_drag).';
Torques = (T_buoy + T_tail + [T_roll_pec; T_pitch_pec; 0] + T_dorsal + T_rot_damp).';


end

== matlab function DolphinDrone_backup/AttitudeController/YawWrap ==
  data: e input; y output
function y = YawWrap(e)
%#codegen
y = atan2(sin(e), cos(e));
